simulink model "n98tot98reg60neu"  (R2023b)
settings: Solver=VariableStepAuto  StartTime=0.0  StopTime=10.0  RelTol=1e-3
libraries: neural x66
(part 2 of 3)

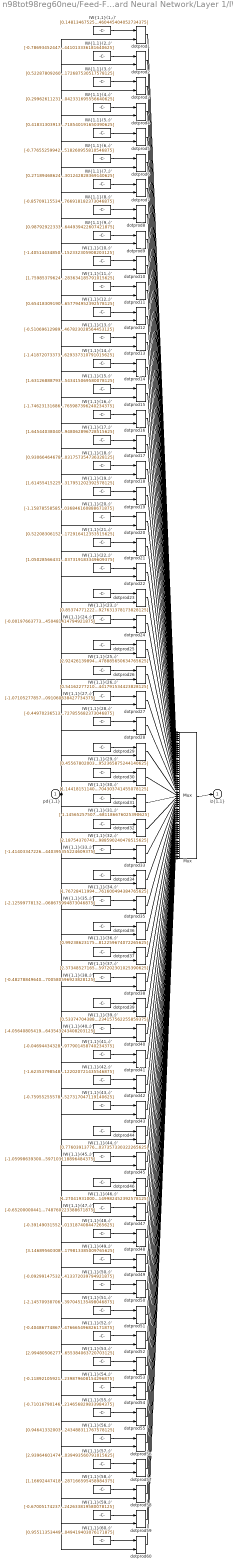
== system n98tot98reg60neu/Feed-Forward Neural Network/Layer 1/IW{1,1} ==
  "pd{1,1}" : Inport  PortDimensions=7
      mask Display: e = 0.06;c1 = [120 230 180]/255;c2 = ([120 230 180]+0)/(256+128);c3 = ([120 230 180]+128)/(256+128);patch([0 1 1 0],[0 0 1 1],c1);patch([0 1 1 1-e 1-e 0+e],[0 0 1 1-e 0+e 0+e],c2);patch([0 0 1 1-e 0+e 0+e],[0 1 1 1-e 1-e 0+e],c3);plot([0 1 1 0 0],[0 0 1 1 0]);
  "IW{1,1}(1,:)'" : Constant  Value=[0.1481346752533242161486981558482511900365352630615234375;0.98082353054952253756937352591194212436676025390625;-2.082918281795799853028938741772435605525970458984375;0.40694944026411672410858955117873847484588623046875;-1.0518399557692712509293642142438329756259918212890625;1.2557149846669120041298128853668458759784698486328125;-0.67808270069946752212075580246164463460445404052734375]
      mask Display: e = 0.06;c1 = [120 150 230]/255;c2 = ([120 150 230]+0)/383;c3 = ([120 150 230]+128)/383;patch([0 1 1 0],[0 0 1 1],c1);patch([0 1 1 1-e 1-e 0+e],[0 0 1 1-e 0+e 0+e],c2);patch([0 0 1 1-e 0+e 0+e],[0 1 1 1-e 1-e 0+e],c3);plot([0 1 1 0 0],[0 0 1 1 0]);disp('Weights');
  "IW{1,1}(10,:)'" : Constant  Value=[-1.4051443485085826079483695139060728251934051513671875;0.487311062264708161340109882075921632349491119384765625;-0.9939232561735884541320729113067500293254852294921875;0.69193945193100725443713372442289255559444427490234375;2.418400242942244648958194375154562294483184814453125;-3.03067098031489390308479414670728147029876708984375;-1.6729437161008047230126294380170293152332305908203125]
      mask Display: e = 0.06;c1 = [120 150 230]/255;c2 = ([120 150 230]+0)/383;c3 = ([120 150 230]+128)/383;patch([0 1 1 0],[0 0 1 1],c1);patch([0 1 1 1-e 1-e 0+e],[0 0 1 1-e 0+e 0+e],c2);patch([0 0 1 1-e 0+e 0+e],[0 1 1 1-e 1-e 0+e],c3);plot([0 1 1 0 0],[0 0 1 1 0]);disp('Weights');
  "IW{1,1}(11,:)'" : Constant  Value=[1.759853796240600676270560143166221678256988525390625;-0.55894441450671905613489798270165920257568359375;-1.4532069951682655695179846588871441781520843505859375;-1.18865973477518327428015254554338753223419189453125;0.89752928329863934653332080415566451847553253173828125;1.1526682692309073718917034057085402309894561767578125;-1.1487702266456720767706656260997988283634185791015625]
      mask Display: e = 0.06;c1 = [120 150 230]/255;c2 = ([120 150 230]+0)/383;c3 = ([120 150 230]+128)/383;patch([0 1 1 0],[0 0 1 1],c1);patch([0 1 1 1-e 1-e 0+e],[0 0 1 1-e 0+e 0+e],c2);patch([0 0 1 1-e 0+e 0+e],[0 1 1 1-e 1-e 0+e],c3);plot([0 1 1 0 0],[0 0 1 1 0]);disp('Weights');
  "IW{1,1}(12,:)'" : Constant  Value=[0.6541830919058633231344401792739517986774444580078125;-0.98785279841036466308423769078217446804046630859375;0.5520966690451316605248166524688713252544403076171875;-0.417983555830826636334762724800384603440761566162109375;-0.9204938395589810085084536694921553134918212890625;0.93854167778469499427984601425123400986194610595703125;-0.469771047647070283392878309314255602657794952392578125]
      mask Display: e = 0.06;c1 = [120 150 230]/255;c2 = ([120 150 230]+0)/383;c3 = ([120 150 230]+128)/383;patch([0 1 1 0],[0 0 1 1],c1);patch([0 1 1 1-e 1-e 0+e],[0 0 1 1-e 0+e 0+e],c2);patch([0 0 1 1-e 0+e 0+e],[0 1 1 1-e 1-e 0+e],c3);plot([0 1 1 0 0],[0 0 1 1 0]);disp('Weights');
  "IW{1,1}(13,:)'" : Constant  Value=[-0.51069612989874146879998306758352555334568023681640625;0.412856570783323884032967043822281993925571441650390625;0.397626390946691110617194908627425320446491241455078125;0.0344230577253679115301565616391599178314208984375;1.03739130513506427888614780385978519916534423828125;0.92439008882190598637151879302109591662883758544921875;0.03278356001701394906167053022727486677467823028564453125]
      mask Display: e = 0.06;c1 = [120 150 230]/255;c2 = ([120 150 230]+0)/383;c3 = ([120 150 230]+128)/383;patch([0 1 1 0],[0 0 1 1],c1);patch([0 1 1 1-e 1-e 0+e],[0 0 1 1-e 0+e 0+e],c2);patch([0 0 1 1-e 0+e 0+e],[0 1 1 1-e 1-e 0+e],c3);plot([0 1 1 0 0],[0 0 1 1 0]);disp('Weights');
  "IW{1,1}(14,:)'" : Constant  Value=[-1.4187207337306324550496583469794131815433502197265625;-0.431927417827714654752213618849054910242557525634765625;0.152434941407513291355968476636917330324649810791015625;-2.027428553931468702131724057835526764392852783203125;1.3251072881331922292957870013196952641010284423828125;0.6240741942748850856759190719458274543285369873046875;2.084603798637122196169002563692629337310791015625]
      mask Display: e = 0.06;c1 = [120 150 230]/255;c2 = ([120 150 230]+0)/383;c3 = ([120 150 230]+128)/383;patch([0 1 1 0],[0 0 1 1],c1);patch([0 1 1 1-e 1-e 0+e],[0 0 1 1-e 0+e 0+e],c2);patch([0 0 1 1-e 0+e 0+e],[0 1 1 1-e 1-e 0+e],c3);plot([0 1 1 0 0],[0 0 1 1 0]);disp('Weights');
  "IW{1,1}(15,:)'" : Constant  Value=[1.6312688879348937742719272137037478387355804443359375;-1.162534244233608848873018359881825745105743408203125;1.0284685549397938331139812362380325794219970703125;2.455316875408408261449721976532600820064544677734375;-2.869144685433620001191457049571909010410308837890625;1.3375400695654622307273484693723730742931365966796875;2.6889193919281684230782047961838543415069580078125]
      mask Display: e = 0.06;c1 = [120 150 230]/255;c2 = ([120 150 230]+0)/383;c3 = ([120 150 230]+128)/383;patch([0 1 1 0],[0 0 1 1],c1);patch([0 1 1 1-e 1-e 0+e],[0 0 1 1-e 0+e 0+e],c2);patch([0 0 1 1-e 0+e 0+e],[0 1 1 1-e 1-e 0+e],c3);plot([0 1 1 0 0],[0 0 1 1 0]);disp('Weights');
  "IW{1,1}(16,:)'" : Constant  Value=[-1.746231316863945171036220926907844841480255126953125;-1.15887605284371719704950010054744780063629150390625;0.50001076713111769489472635541460476815700531005859375;-2.84379068119553313209735279087908565998077392578125;0.129001045300250638536709857362438924610614776611328125;-1.0933162048887756778725588446832261979579925537109375;0.7263530548743071246775571125908754765987396240234375]
      mask Display: e = 0.06;c1 = [120 150 230]/255;c2 = ([120 150 230]+0)/383;c3 = ([120 150 230]+128)/383;patch([0 1 1 0],[0 0 1 1],c1);patch([0 1 1 1-e 1-e 0+e],[0 0 1 1-e 0+e 0+e],c2);patch([0 0 1 1-e 0+e 0+e],[0 1 1 1-e 1-e 0+e],c3);plot([0 1 1 0 0],[0 0 1 1 0]);disp('Weights');
  "IW{1,1}(17,:)'" : Constant  Value=[1.64544038040287698976271713036112487316131591796875;-3.633653677731499609393495120457373559474945068359375;-2.29787262698807293048730571172200143337249755859375;0.078067342091915847834826536200125701725482940673828125;-0.577295747878546539055832909070886671543121337890625;-1.619702917064653302503529630484990775585174560546875;1.7761068046404473452781758169294334948062896728515625]
      mask Display: e = 0.06;c1 = [120 150 230]/255;c2 = ([120 150 230]+0)/383;c3 = ([120 150 230]+128)/383;patch([0 1 1 0],[0 0 1 1],c1);patch([0 1 1 1-e 1-e 0+e],[0 0 1 1-e 0+e 0+e],c2);patch([0 0 1 1-e 0+e 0+e],[0 1 1 1-e 1-e 0+e],c3);plot([0 1 1 0 0],[0 0 1 1 0]);disp('Weights');
  "IW{1,1}(18,:)'" : Constant  Value=[0.93066464678121019193923757484299130737781524658203125;-1.9544287349273126164206360044772736728191375732421875;-1.023472620127600318795657585724256932735443115234375;0.98793022766258375977344030616222880780696868896484375;1.6281013571460698496906616128399036824703216552734375;-0.0185687723603052794174583794983846019022166728973388671875;-0.2930769639165078377374129559029825031757354736328125]
      mask Display: e = 0.06;c1 = [120 150 230]/255;c2 = ([120 150 230]+0)/383;c3 = ([120 150 230]+128)/383;patch([0 1 1 0],[0 0 1 1],c1);patch([0 1 1 1-e 1-e 0+e],[0 0 1 1-e 0+e 0+e],c2);patch([0 0 1 1-e 0+e 0+e],[0 1 1 1-e 1-e 0+e],c3);plot([0 1 1 0 0],[0 0 1 1 0]);disp('Weights');
  "IW{1,1}(19,:)'" : Constant  Value=[1.6145541522585509230935940649942494928836822509765625;0.91381367394026347117375053130672313272953033447265625;-0.371631548982591042307177531256456859409809112548828125;0.73502527154724550673137173362192697823047637939453125;1.5056615216127851031302498086006380617618560791015625;1.15739385289584983951272079139016568660736083984375;-1.45708523863142591636687939171679317951202392578125]
      mask Display: e = 0.06;c1 = [120 150 230]/255;c2 = ([120 150 230]+0)/383;c3 = ([120 150 230]+128)/383;patch([0 1 1 0],[0 0 1 1],c1);patch([0 1 1 1-e 1-e 0+e],[0 0 1 1-e 0+e 0+e],c2);patch([0 0 1 1-e 0+e 0+e],[0 1 1 1-e 1-e 0+e],c3);plot([0 1 1 0 0],[0 0 1 1 0]);disp('Weights');
  "IW{1,1}(2,:)'" : Constant  Value=[-0.7869345244760317381604863840038888156414031982421875;-0.346311954352809092672060842232895083725452423095703125;-1.556955762008559229769844023394398391246795654296875;-0.51529864332368091606184634656528942286968231201171875;0.868254630896831969266713713295757770538330078125;0.052275095673093983916768223707549623213708400726318359375;1.454283513794509818950473345466889441013336181640625]
      mask Display: e = 0.06;c1 = [120 150 230]/255;c2 = ([120 150 230]+0)/383;c3 = ([120 150 230]+128)/383;patch([0 1 1 0],[0 0 1 1],c1);patch([0 1 1 1-e 1-e 0+e],[0 0 1 1-e 0+e 0+e],c2);patch([0 0 1 1-e 0+e 0+e],[0 1 1 1-e 1-e 0+e],c3);plot([0 1 1 0 0],[0 0 1 1 0]);disp('Weights');
  "IW{1,1}(20,:)'" : Constant  Value=[-1.158785585859792188756500763702206313610076904296875;-0.9101893538308860609475914316135458648204803466796875;-0.2242153799095476240932356404300662688910961151123046875;4.6125770809612678391431472846306860446929931640625;-1.967721084439806755739255095249973237514495849609375;0.77232129956188710906417327350936830043792724609375;-0.07051684698582198762562001093101571314036846160888671875]
      mask Display: e = 0.06;c1 = [120 150 230]/255;c2 = ([120 150 230]+0)/383;c3 = ([120 150 230]+128)/383;patch([0 1 1 0],[0 0 1 1],c1);patch([0 1 1 1-e 1-e 0+e],[0 0 1 1-e 0+e 0+e],c2);patch([0 0 1 1-e 0+e 0+e],[0 1 1 1-e 1-e 0+e],c3);plot([0 1 1 0 0],[0 0 1 1 0]);disp('Weights');
  "IW{1,1}(21,:)'" : Constant  Value=[0.52208306152979744307884857335011474788188934326171875;-0.24553627119159637803846862880163826048374176025390625;0.74283311097407267453718304750509560108184814453125;-0.8132083009806365669902561421622522175312042236328125;-1.6353310904372870826506414232426322996616363525390625;0.804047841179728717264652004814706742763519287109375;0.30147537024770498792491935091675259172916412353515625]
      mask Display: e = 0.06;c1 = [120 150 230]/255;c2 = ([120 150 230]+0)/383;c3 = ([120 150 230]+128)/383;patch([0 1 1 0],[0 0 1 1],c1);patch([0 1 1 1-e 1-e 0+e],[0 0 1 1-e 0+e 0+e],c2);patch([0 0 1 1-e 0+e 0+e],[0 1 1 1-e 1-e 0+e],c3);plot([0 1 1 0 0],[0 0 1 1 0]);disp('Weights');
  "IW{1,1}(22,:)'" : Constant  Value=[1.050285664310628863660213028197176754474639892578125;-0.1436604121479605200573104184513795189559459686279296875;1.3658699547684276520698176682344637811183929443359375;-2.139623131427094815393274984671734273433685302734375;-0.476115789654785681594972857055836357176303863525390625;-2.445497663519104580842622453928925096988677978515625;-0.95852873762775236965438807601458393037319183349609375]
      mask Display: e = 0.06;c1 = [120 150 230]/255;c2 = ([120 150 230]+0)/383;c3 = ([120 150 230]+128)/383;patch([0 1 1 0],[0 0 1 1],c1);patch([0 1 1 1-e 1-e 0+e],[0 0 1 1-e 0+e 0+e],c2);patch([0 0 1 1-e 0+e 0+e],[0 1 1 1-e 1-e 0+e],c3);plot([0 1 1 0 0],[0 0 1 1 0]);disp('Weights');
  "IW{1,1}(23,:)'" : Constant  Value=[0.85374771222291812033944324866752140223979949951171875;1.4611201108056064423834641274879686534404754638671875;-0.71512999345489658420405021388432942330837249755859375;-1.5360765778745673060257104225456714630126953125;1.3057858257014036684751090433564968407154083251953125;-1.0436475254304660165161067197914235293865203857421875;1.2728096477339807535145155270583927631378173828125]
      mask Display: e = 0.06;c1 = [120 150 230]/255;c2 = ([120 150 230]+0)/383;c3 = ([120 150 230]+128)/383;patch([0 1 1 0],[0 0 1 1],c1);patch([0 1 1 1-e 1-e 0+e],[0 0 1 1-e 0+e 0+e],c2);patch([0 0 1 1-e 0+e 0+e],[0 1 1 1-e 1-e 0+e],c3);plot([0 1 1 0 0],[0 0 1 1 0]);disp('Weights');
  "IW{1,1}(24,:)'" : Constant  Value=[-0.0019766377326448647533396751896361820399761199951171875;-0.83118616146239043818155778353684581816196441650390625;0.373888659074529117187779547748505137860774993896484375;1.59975498434179375095709474408067762851715087890625;1.8936310356371277574538680710247717797756195068359375;-2.56484219821481662648920973879285156726837158203125;-0.73221593302772880473838768011773936450481414794921875]
      mask Display: e = 0.06;c1 = [120 150 230]/255;c2 = ([120 150 230]+0)/383;c3 = ([120 150 230]+128)/383;patch([0 1 1 0],[0 0 1 1],c1);patch([0 1 1 1-e 1-e 0+e],[0 0 1 1-e 0+e 0+e],c2);patch([0 0 1 1-e 0+e 0+e],[0 1 1 1-e 1-e 0+e],c3);plot([0 1 1 0 0],[0 0 1 1 0]);disp('Weights');
  "IW{1,1}(25,:)'" : Constant  Value=[2.924261398940739553609091672115027904510498046875;1.01135703353342254473545835935510694980621337890625;-0.40057513886989604134925002654199488461017608642578125;1.117845219342571194687252500443719327449798583984375;1.487336953128143068880717692081816494464874267578125;-0.3337818787676083420734585160971619188785552978515625;3.366286632630610231586842928663827478885650634765625]
      mask Display: e = 0.06;c1 = [120 150 230]/255;c2 = ([120 150 230]+0)/383;c3 = ([120 150 230]+128)/383;patch([0 1 1 0],[0 0 1 1],c1);patch([0 1 1 1-e 1-e 0+e],[0 0 1 1-e 0+e 0+e],c2);patch([0 0 1 1-e 0+e 0+e],[0 1 1 1-e 1-e 0+e],c3);plot([0 1 1 0 0],[0 0 1 1 0]);disp('Weights');
  "IW{1,1}(26,:)'" : Constant  Value=[0.54162277210162113050273546832613646984100341796875;0.456056013547237182326199445014935918152332305908203125;1.4394577727029942426639763652929104864597320556640625;0.58974019201134175727219144391710869967937469482421875;1.9862617127959680818349852415849454700946807861328125;0.291103928669838751819298749978770501911640167236328125;-2.381474711015628020760459548910148441791534423828125]
      mask Display: e = 0.06;c1 = [120 150 230]/255;c2 = ([120 150 230]+0)/383;c3 = ([120 150 230]+128)/383;patch([0 1 1 0],[0 0 1 1],c1);patch([0 1 1 1-e 1-e 0+e],[0 0 1 1-e 0+e 0+e],c2);patch([0 0 1 1-e 0+e 0+e],[0 1 1 1-e 1-e 0+e],c3);plot([0 1 1 0 0],[0 0 1 1 0]);disp('Weights');
  "IW{1,1}(27,:)'" : Constant  Value=[-1.071052778571999652967861038632690906524658203125;-2.02899035921602344245684435009025037288665771484375;-0.8560859121211625843983483719057403504848480224609375;0.59540640519818233133975127202575094997882843017578125;0.75214105415422505274136710795573890209197998046875;-0.43346848639706792027936899103224277496337890625;1.076762221099778482624742537154816091060638427734375]
      mask Display: e = 0.06;c1 = [120 150 230]/255;c2 = ([120 150 230]+0)/383;c3 = ([120 150 230]+128)/383;patch([0 1 1 0],[0 0 1 1],c1);patch([0 1 1 1-e 1-e 0+e],[0 0 1 1-e 0+e 0+e],c2);patch([0 0 1 1-e 0+e 0+e],[0 1 1 1-e 1-e 0+e],c3);plot([0 1 1 0 0],[0 0 1 1 0]);disp('Weights');
  "IW{1,1}(28,:)'" : Constant  Value=[-0.4497023651390212872769325258559547364711761474609375;-0.8805125386607233206603950748103670775890350341796875;-1.606489318533170784775165884639136493206024169921875;-1.447323751073491759910893961205147206783294677734375;1.3204566033571929484224938278202898800373077392578125;-0.1433022562635145880083342717625782825052738189697265625;-1.173633507304539858040470790001563727855682373046875]
      mask Display: e = 0.06;c1 = [120 150 230]/255;c2 = ([120 150 230]+0)/383;c3 = ([120 150 230]+128)/383;patch([0 1 1 0],[0 0 1 1],c1);patch([0 1 1 1-e 1-e 0+e],[0 0 1 1-e 0+e 0+e],c2);patch([0 0 1 1-e 0+e 0+e],[0 1 1 1-e 1-e 0+e],c3);plot([0 1 1 0 0],[0 0 1 1 0]);disp('Weights');
  "IW{1,1}(29,:)'" : Constant  Value=[0.455678020034327946330421355014550499618053436279296875;1.0449829035940758625855551144923083484172821044921875;-2.051400565385125940309762881952337920665740966796875;-2.269241494744366871572083255159668624401092529296875;4.0322839793207787550954890321008861064910888671875;0.80328637261176349948499364472809247672557830810546875;4.19454985578971051296548466780222952365875244140625]
      mask Display: e = 0.06;c1 = [120 150 230]/255;c2 = ([120 150 230]+0)/383;c3 = ([120 150 230]+128)/383;patch([0 1 1 0],[0 0 1 1],c1);patch([0 1 1 1-e 1-e 0+e],[0 0 1 1-e 0+e 0+e],c2);patch([0 0 1 1-e 0+e 0+e],[0 1 1 1-e 1-e 0+e],c3);plot([0 1 1 0 0],[0 0 1 1 0]);disp('Weights');
  "IW{1,1}(3,:)'" : Constant  Value=[0.52287809260233941710538374536554329097270965576171875;0.355086158017595965308288441519835032522678375244140625;0.3211806987072407526540018807281740009784698486328125;-0.172433039949836774962221852547372691333293914794921875;-0.02907109420287723455800232841284014284610748291015625;-0.936005019789345027447780012153089046478271484375;1.1683911275902467696852227163617499172687530517578125]
      mask Display: e = 0.06;c1 = [120 150 230]/255;c2 = ([120 150 230]+0)/383;c3 = ([120 150 230]+128)/383;patch([0 1 1 0],[0 0 1 1],c1);patch([0 1 1 1-e 1-e 0+e],[0 0 1 1-e 0+e 0+e],c2);patch([0 0 1 1-e 0+e 0+e],[0 1 1 1-e 1-e 0+e],c3);plot([0 1 1 0 0],[0 0 1 1 0]);disp('Weights');
  "IW{1,1}(30,:)'" : Constant  Value=[1.1441815114008682119361992590711452066898345947265625;0.02635002074122540227651967370547936297953128814697265625;1.1697060189576917732523497761576436460018157958984375;-2.07603958112650044398606041795574128627777099609375;-1.523338123097244700687724616727791726589202880859375;1.2813465289053180828915401434642262756824493408203125;-0.301678114240235828447111998684704303741455078125]
      mask Display: e = 0.06;c1 = [120 150 230]/255;c2 = ([120 150 230]+0)/383;c3 = ([120 150 230]+128)/383;patch([0 1 1 0],[0 0 1 1],c1);patch([0 1 1 1-e 1-e 0+e],[0 0 1 1-e 0+e 0+e],c2);patch([0 0 1 1-e 0+e 0+e],[0 1 1 1-e 1-e 0+e],c3);plot([0 1 1 0 0],[0 0 1 1 0]);disp('Weights');
  "IW{1,1}(31,:)'" : Constant  Value=[-1.1456525750787356354720714080031029880046844482421875;-0.301316378862511335956497759980265982449054718017578125;-0.6999713143398993420163378686993382871150970458984375;-1.888670407036998621919110519229434430599212646484375;-0.51493465015129358253176405924023129045963287353515625;1.09374415185767315250586761976592242717742919921875;-1.172688349926057416183766690664924681186676025390625]
      mask Display: e = 0.06;c1 = [120 150 230]/255;c2 = ([120 150 230]+0)/383;c3 = ([120 150 230]+128)/383;patch([0 1 1 0],[0 0 1 1],c1);patch([0 1 1 1-e 1-e 0+e],[0 0 1 1-e 0+e 0+e],c2);patch([0 0 1 1-e 0+e 0+e],[0 1 1 1-e 1-e 0+e],c3);plot([0 1 1 0 0],[0 0 1 1 0]);disp('Weights');
  "IW{1,1}(32,:)'" : Constant  Value=[2.187543707432160200454518417245708405971527099609375;0.7832629532967370078466728955390863120555877685546875;0.97277406417956502338029167731292545795440673828125;0.169364411870373654522836659452877938747406005859375;-0.1872178173399863532200271265537594445049762725830078125;-1.635072077562477854684175326838158071041107177734375;0.0374795167828784470120950800264836288988590240478515625]
      mask Display: e = 0.06;c1 = [120 150 230]/255;c2 = ([120 150 230]+0)/383;c3 = ([120 150 230]+128)/383;patch([0 1 1 0],[0 0 1 1],c1);patch([0 1 1 1-e 1-e 0+e],[0 0 1 1-e 0+e 0+e],c2);patch([0 0 1 1-e 0+e 0+e],[0 1 1 1-e 1-e 0+e],c3);plot([0 1 1 0 0],[0 0 1 1 0]);disp('Weights');
  "IW{1,1}(33,:)'" : Constant  Value=[-1.4140334722618492779844245887943543493747711181640625;-1.066226188394075347076750404085032641887664794921875;-0.74303173177076786704020605611731298267841339111328125;0.59865982615122026455622972207493148744106292724609375;-0.46737583966662021861537823497201316058635711669921875;-0.145915447642352480439598139128065668046474456787109375;0.6450607346262733354791407691664062440395355224609375]
      mask Display: e = 0.06;c1 = [120 150 230]/255;c2 = ([120 150 230]+0)/383;c3 = ([120 150 230]+128)/383;patch([0 1 1 0],[0 0 1 1],c1);patch([0 1 1 1-e 1-e 0+e],[0 0 1 1-e 0+e 0+e],c2);patch([0 0 1 1-e 0+e 0+e],[0 1 1 1-e 1-e 0+e],c3);plot([0 1 1 0 0],[0 0 1 1 0]);disp('Weights');
  "IW{1,1}(34,:)'" : Constant  Value=[1.767284119945664588868794453446753323078155517578125;-0.6493741207138825632938505805213935673236846923828125;-0.255236564518358355346805410590604878962039947509765625;-2.13669533467837791107513112365268170833587646484375;0.80266841289320833841003377528977580368518829345703125;0.61122329910277761744197277948842383921146392822265625;-0.5399939366629686876564164776937104761600494384765625]
      mask Display: e = 0.06;c1 = [120 150 230]/255;c2 = ([120 150 230]+0)/383;c3 = ([120 150 230]+128)/383;patch([0 1 1 0],[0 0 1 1],c1);patch([0 1 1 1-e 1-e 0+e],[0 0 1 1-e 0+e 0+e],c2);patch([0 0 1 1-e 0+e 0+e],[0 1 1 1-e 1-e 0+e],c3);plot([0 1 1 0 0],[0 0 1 1 0]);disp('Weights');
  "IW{1,1}(35,:)'" : Constant  Value=[-2.12599778132206562730743826250545680522918701171875;1.3608125008815721290744704674580134451389312744140625;-0.7325358825414862717906316902372054755687713623046875;0.240060365986900781098967172511038370430469512939453125;0.18982699817795001262510368178482167422771453857421875;-1.0066882538136978642029362163157202303409576416015625;0.667860286161154004247464399668388068675994873046875]
      mask Display: e = 0.06;c1 = [120 150 230]/255;c2 = ([120 150 230]+0)/383;c3 = ([120 150 230]+128)/383;patch([0 1 1 0],[0 0 1 1],c1);patch([0 1 1 1-e 1-e 0+e],[0 0 1 1-e 0+e 0+e],c2);patch([0 0 1 1-e 0+e 0+e],[0 1 1 1-e 1-e 0+e],c3);plot([0 1 1 0 0],[0 0 1 1 0]);disp('Weights');
  "IW{1,1}(36,:)'" : Constant  Value=[0.992386231759784909201016489532776176929473876953125;-0.10079863677393478826882500243300455622375011444091796875;-0.89913155892687812720254214582382701337337493896484375;-1.153666025787317916950769358663819730281829833984375;0.186564489102124586583641985271242447197437286376953125;2.13673253963647180597718033823184669017791748046875;2.591152548548058209831879139528609812259674072265625]
      mask Display: e = 0.06;c1 = [120 150 230]/255;c2 = ([120 150 230]+0)/383;c3 = ([120 150 230]+128)/383;patch([0 1 1 0],[0 0 1 1],c1);patch([0 1 1 1-e 1-e 0+e],[0 0 1 1-e 0+e 0+e],c2);patch([0 0 1 1-e 0+e 0+e],[0 1 1 1-e 1-e 0+e],c3);plot([0 1 1 0 0],[0 0 1 1 0]);disp('Weights');
  "IW{1,1}(37,:)'" : Constant  Value=[2.373485271659477202632615444599650800228118896484375;-2.83140944472043454283038954599760472774505615234375;-0.2381591970668265056954027159008546732366085052490234375;1.6073649182960274561793312386726029217243194580078125;0.1270632058802902975003235042095184326171875;-0.290937777914213047125713273999281227588653564453125;2.903333553776429543091808227472938597202301025390625]
      mask Display: e = 0.06;c1 = [120 150 230]/255;c2 = ([120 150 230]+0)/383;c3 = ([120 150 230]+128)/383;patch([0 1 1 0],[0 0 1 1],c1);patch([0 1 1 1-e 1-e 0+e],[0 0 1 1-e 0+e 0+e],c2);patch([0 0 1 1-e 0+e 0+e],[0 1 1 1-e 1-e 0+e],c3);plot([0 1 1 0 0],[0 0 1 1 0]);disp('Weights');
  "IW{1,1}(38,:)'" : Constant  Value=[-0.482788496408222689293410212485468946397304534912109375;1.6104028950399194020093318613362498581409454345703125;-1.865988325170027994914789815084077417850494384765625;0.75686623013146536731454716573352925479412078857421875;0.803638662707797823969713135738857090473175048828125;-0.624867558425080016348829303751699626445770263671875;0.73596606492041971581130610502441413700580596923828125]
      mask Display: e = 0.06;c1 = [120 150 230]/255;c2 = ([120 150 230]+0)/383;c3 = ([120 150 230]+128)/383;patch([0 1 1 0],[0 0 1 1],c1);patch([0 1 1 1-e 1-e 0+e],[0 0 1 1-e 0+e 0+e],c2);patch([0 0 1 1-e 0+e 0+e],[0 1 1 1-e 1-e 0+e],c3);plot([0 1 1 0 0],[0 0 1 1 0]);disp('Weights');
  "IW{1,1}(39,:)'" : Constant  Value=[0.5337470438813813888856429912266321480274200439453125;0.84274856967459876866399781647487543523311614990234375;-1.95409080267971635436197175295092165470123291015625;0.42544403042022604921612582984380424022674560546875;0.9690675152028200844966931981616653501987457275390625;0.0163222485195519372014327785791465430520474910736083984375;-0.491484984158165827405895242918631993234157562255859375]
      mask Display: e = 0.06;c1 = [120 150 230]/255;c2 = ([120 150 230]+0)/383;c3 = ([120 150 230]+128)/383;patch([0 1 1 0],[0 0 1 1],c1);patch([0 1 1 1-e 1-e 0+e],[0 0 1 1-e 0+e 0+e],c2);patch([0 0 1 1-e 0+e 0+e],[0 1 1 1-e 1-e 0+e],c3);plot([0 1 1 0 0],[0 0 1 1 0]);disp('Weights');
  "IW{1,1}(4,:)'" : Constant  Value=[0.299626112316270176716415107875945977866649627685546875;-0.044314293017502691396369840504121384583413600921630859375;-0.8841463713183135286755032211658544838428497314453125;0.7744232725463380262453938485123217105865478515625;1.8909629644727130592940511633059941232204437255859375;0.062323560497111706035777700662947609089314937591552734375;-0.11719207511177499869692297806977876462042331695556640625]
      mask Display: e = 0.06;c1 = [120 150 230]/255;c2 = ([120 150 230]+0)/383;c3 = ([120 150 230]+128)/383;patch([0 1 1 0],[0 0 1 1],c1);patch([0 1 1 1-e 1-e 0+e],[0 0 1 1-e 0+e 0+e],c2);patch([0 0 1 1-e 0+e 0+e],[0 1 1 1-e 1-e 0+e],c3);plot([0 1 1 0 0],[0 0 1 1 0]);disp('Weights');
  "IW{1,1}(40,:)'" : Constant  Value=[-4.05640805419469785420005791820585727691650390625;0.0873765616747470830194544078040053136646747589111328125;0.54901834404562188662879407274886034429073333740234375;0.89968084756964561421455073286779224872589111328125;1.7184637967256561896789435195387341082096099853515625;-1.3935197143518334161882421540212817490100860595703125;-2.623692509614226953118532037478871643543243408203125]
      mask Display: e = 0.06;c1 = [120 150 230]/255;c2 = ([120 150 230]+0)/383;c3 = ([120 150 230]+128)/383;patch([0 1 1 0],[0 0 1 1],c1);patch([0 1 1 1-e 1-e 0+e],[0 0 1 1-e 0+e 0+e],c2);patch([0 0 1 1-e 0+e 0+e],[0 1 1 1-e 1-e 0+e],c3);plot([0 1 1 0 0],[0 0 1 1 0]);disp('Weights');
  "IW{1,1}(41,:)'" : Constant  Value=[-0.046944343288031924188441479373068432323634624481201171875;-2.21537331420981953300497480086050927639007568359375;-1.2718477750401888659581572937895543873310089111328125;0.2532434280552477989800763680250383913516998291015625;-0.38837008773848669118677889855462126433849334716796875;1.0430562979632067577284715298446826636791229248046875;-0.92779194210217408311791587038896977901458740234375]
      mask Display: e = 0.06;c1 = [120 150 230]/255;c2 = ([120 150 230]+0)/383;c3 = ([120 150 230]+128)/383;patch([0 1 1 0],[0 0 1 1],c1);patch([0 1 1 1-e 1-e 0+e],[0 0 1 1-e 0+e 0+e],c2);patch([0 0 1 1-e 0+e 0+e],[0 1 1 1-e 1-e 0+e],c3);plot([0 1 1 0 0],[0 0 1 1 0]);disp('Weights');
  "IW{1,1}(42,:)'" : Constant  Value=[-1.6235379854818445810593630085350014269351959228515625;0.98250437107865373764781224963371641933917999267578125;1.90239772700385589843108391505666077136993408203125;0.3618940465058153588273626155569218099117279052734375;0.311560429313485542923700677420129068195819854736328125;2.113010718428258716272694073268212378025054931640625;-0.08559181635963357404062179512038710527122020721435546875]
      mask Display: e = 0.06;c1 = [120 150 230]/255;c2 = ([120 150 230]+0)/383;c3 = ([120 150 230]+128)/383;patch([0 1 1 0],[0 0 1 1],c1);patch([0 1 1 1-e 1-e 0+e],[0 0 1 1-e 0+e 0+e],c2);patch([0 0 1 1-e 0+e 0+e],[0 1 1 1-e 1-e 0+e],c3);plot([0 1 1 0 0],[0 0 1 1 0]);disp('Weights');
  "IW{1,1}(43,:)'" : Constant  Value=[-0.75955255578861358145559279364533722400665283203125;1.3921115451136893970129904118948616087436676025390625;0.438296223731076184382260407801368273794651031494140625;-0.78872599627513484410457067497191019356250762939453125;-1.7965397122145831954043160294531844556331634521484375;0.41442701575381268863651484934962354600429534912109375;-0.7917432291391934828794774148263968527317047119140625]
      mask Display: e = 0.06;c1 = [120 150 230]/255;c2 = ([120 150 230]+0)/383;c3 = ([120 150 230]+128)/383;patch([0 1 1 0],[0 0 1 1],c1);patch([0 1 1 1-e 1-e 0+e],[0 0 1 1-e 0+e 0+e],c2);patch([0 0 1 1-e 0+e 0+e],[0 1 1 1-e 1-e 0+e],c3);plot([0 1 1 0 0],[0 0 1 1 0]);disp('Weights');
  "IW{1,1}(44,:)'" : Constant  Value=[0.77603913776969035698272136869491077959537506103515625;1.68618633989586275134797688224352896213531494140625;-0.0668610125904696150911377117154188454151153564453125;-0.54391986928281832458509370553656481206417083740234375;-1.628652778124873190535026878933422267436981201171875;1.319361974881373189560918035567738115787506103515625;-1.025986300680023166620458141551353037357330322265625]
      mask Display: e = 0.06;c1 = [120 150 230]/255;c2 = ([120 150 230]+0)/383;c3 = ([120 150 230]+128)/383;patch([0 1 1 0],[0 0 1 1],c1);patch([0 1 1 1-e 1-e 0+e],[0 0 1 1-e 0+e 0+e],c2);patch([0 0 1 1-e 0+e 0+e],[0 1 1 1-e 1-e 0+e],c3);plot([0 1 1 0 0],[0 0 1 1 0]);disp('Weights');
  "IW{1,1}(45,:)'" : Constant  Value=[-1.059986393001422388948640218586660921573638916015625;-0.173101130652922263752913067946792580187320709228515625;0.5844790773023811336628341450705192983150482177734375;-1.4850851960119795247550200656405650079250335693359375;-2.491597453765368896938525722362101078033447265625;-0.69934109868302651857874252527835778892040252685546875;-0.9044014878802657531053910133778117597103118896484375]
      mask Display: e = 0.06;c1 = [120 150 230]/255;c2 = ([120 150 230]+0)/383;c3 = ([120 150 230]+128)/383;patch([0 1 1 0],[0 0 1 1],c1);patch([0 1 1 1-e 1-e 0+e],[0 0 1 1-e 0+e 0+e],c2);patch([0 0 1 1-e 0+e 0+e],[0 1 1 1-e 1-e 0+e],c3);plot([0 1 1 0 0],[0 0 1 1 0]);disp('Weights');
  "IW{1,1}(46,:)'" : Constant  Value=[1.2704193100027347806957322973175905644893646240234375;0.36762899058214071335015660224598832428455352783203125;1.2338475706229130590685372226289473474025726318359375;1.61977613534372721915133297443389892578125;1.4297303052058583094918731148936785757541656494140625;1.009376369554987551424574121483601629734039306640625;-1.5254997695976364457948193376068957149982452392578125]
      mask Display: e = 0.06;c1 = [120 150 230]/255;c2 = ([120 150 230]+0)/383;c3 = ([120 150 230]+128)/383;patch([0 1 1 0],[0 0 1 1],c1);patch([0 1 1 1-e 1-e 0+e],[0 0 1 1-e 0+e 0+e],c2);patch([0 0 1 1-e 0+e 0+e],[0 1 1 1-e 1-e 0+e],c3);plot([0 1 1 0 0],[0 0 1 1 0]);disp('Weights');
  "IW{1,1}(47,:)'" : Constant  Value=[-0.6520000044181470943982503740699030458927154541015625;-2.14807689392080902734960545785725116729736328125;0.30508269178191227410934516228735446929931640625;1.4101409733411525149193721517804078757762908935546875;0.86058815026270452097634233723510988056659698486328125;0.56656820153376930004895939418929629027843475341796875;0.503688223996419548456060510943643748760223388671875]
      mask Display: e = 0.06;c1 = [120 150 230]/255;c2 = ([120 150 230]+0)/383;c3 = ([120 150 230]+128)/383;patch([0 1 1 0],[0 0 1 1],c1);patch([0 1 1 1-e 1-e 0+e],[0 0 1 1-e 0+e 0+e],c2);patch([0 0 1 1-e 0+e 0+e],[0 1 1 1-e 1-e 0+e],c3);plot([0 1 1 0 0],[0 0 1 1 0]);disp('Weights');
  "IW{1,1}(48,:)'" : Constant  Value=[-0.391490315520112763802984545691288076341152191162109375;-0.1411084660676686919345002024783752858638763427734375;1.215498247946994236912132691941224038600921630859375;-0.01961802326384708139439538854276179336011409759521484375;3.85616003720454525449667926295660436153411865234375;0.52960589523922207977335574469179846346378326416015625;-0.977924126398966198081552647636272013187408447265625]
      mask Display: e = 0.06;c1 = [120 150 230]/255;c2 = ([120 150 230]+0)/383;c3 = ([120 150 230]+128)/383;patch([0 1 1 0],[0 0 1 1],c1);patch([0 1 1 1-e 1-e 0+e],[0 0 1 1-e 0+e 0+e],c2);patch([0 0 1 1-e 0+e 0+e],[0 1 1 1-e 1-e 0+e],c3);plot([0 1 1 0 0],[0 0 1 1 0]);disp('Weights');
  "IW{1,1}(49,:)'" : Constant  Value=[3.146895603083233794450279674492776393890380859375;1.7472349608462358627747335049207322299480438232421875;0.7900047284623408216930329217575490474700927734375;-0.4267675030149826742587038097553886473178863525390625;-1.165080190804833382145488940295763313770294189453125;0.71233753204131355918349299827241338789463043212890625;-1.6692508500826639394887251910404302179813385009765625]
      mask Display: e = 0.06;c1 = [120 150 230]/255;c2 = ([120 150 230]+0)/383;c3 = ([120 150 230]+128)/383;patch([0 1 1 0],[0 0 1 1],c1);patch([0 1 1 1-e 1-e 0+e],[0 0 1 1-e 0+e 0+e],c2);patch([0 0 1 1-e 0+e 0+e],[0 1 1 1-e 1-e 0+e],c3);plot([0 1 1 0 0],[0 0 1 1 0]);disp('Weights');
  "IW{1,1}(5,:)'" : Constant  Value=[0.418313039130509434215809960733167827129364013671875;0.59154140343533090362626580827054567635059356689453125;1.52828163417684503855298316921107470989227294921875;-1.3352094420734068602740762798930518329143524169921875;-0.1773906306009228883713291224921704269945621490478515625;-0.9304403197455177743080412255949340760707855224609375;-0.521077102426085847497461145394481718540191650390625]
      mask Display: e = 0.06;c1 = [120 150 230]/255;c2 = ([120 150 230]+0)/383;c3 = ([120 150 230]+128)/383;patch([0 1 1 0],[0 0 1 1],c1);patch([0 1 1 1-e 1-e 0+e],[0 0 1 1-e 0+e 0+e],c2);patch([0 0 1 1-e 0+e 0+e],[0 1 1 1-e 1-e 0+e],c3);plot([0 1 1 0 0],[0 0 1 1 0]);disp('Weights');
  "IW{1,1}(50,:)'" : Constant  Value=[-0.09299147532523883985522417106039938516914844512939453125;0.2212028814998839021388477021901053376495838165283203125;-1.367502038876399428346530839917249977588653564453125;0.149462870458643148907640352263115346431732177734375;1.43803812210721648767730584950186312198638916015625;-0.56873955080151816776634632333298213779926300048828125;-0.418886678529261480274925588673795573413372039794921875]
      mask Display: e = 0.06;c1 = [120 150 230]/255;c2 = ([120 150 230]+0)/383;c3 = ([120 150 230]+128)/383;patch([0 1 1 0],[0 0 1 1],c1);patch([0 1 1 1-e 1-e 0+e],[0 0 1 1-e 0+e 0+e],c2);patch([0 0 1 1-e 0+e 0+e],[0 1 1 1-e 1-e 0+e],c3);plot([0 1 1 0 0],[0 0 1 1 0]);disp('Weights');
  "IW{1,1}(51,:)'" : Constant  Value=[-2.14570938706170455390065399114973843097686767578125;-0.91149469900424351376244658240466378629207611083984375;0.8098365880171394248776550739421509206295013427734375;1.512309897695889748803210750338621437549591064453125;-0.2119992648588315820035177239333279430866241455078125;-1.0326483768972087862181297168717719614505767822265625;-0.85290627225207937822659687299164943397045135498046875]
      mask Display: e = 0.06;c1 = [120 150 230]/255;c2 = ([120 150 230]+0)/383;c3 = ([120 150 230]+128)/383;patch([0 1 1 0],[0 0 1 1],c1);patch([0 1 1 1-e 1-e 0+e],[0 0 1 1-e 0+e 0+e],c2);patch([0 0 1 1-e 0+e 0+e],[0 1 1 1-e 1-e 0+e],c3);plot([0 1 1 0 0],[0 0 1 1 0]);disp('Weights');
  "IW{1,1}(52,:)'" : Constant  Value=[-0.404867748676235150728786038598627783358097076416015625;-0.42029731151777582898176888193120248615741729736328125;1.299408072829371096901240889565087854862213134765625;1.2308012084313804113122614580788649618625640869140625;0.80657817399877862474255607594386674463748931884765625;-0.4344717411564300579840391947072930634021759033203125;-0.55894690716519235262893516846816055476665496826171875]
      mask Display: e = 0.06;c1 = [120 150 230]/255;c2 = ([120 150 230]+0)/383;c3 = ([120 150 230]+128)/383;patch([0 1 1 0],[0 0 1 1],c1);patch([0 1 1 1-e 1-e 0+e],[0 0 1 1-e 0+e 0+e],c2);patch([0 0 1 1-e 0+e 0+e],[0 1 1 1-e 1-e 0+e],c3);plot([0 1 1 0 0],[0 0 1 1 0]);disp('Weights');
  "IW{1,1}(53,:)'" : Constant  Value=[2.994805062774202664144240770838223397731781005859375;0.00956422219174242298211918722472546505741775035858154296875;-1.8875362364771504086746745088021270930767059326171875;1.17653478225301366677513215108774602413177490234375;-2.8280186048595368220048840157687664031982421875;-0.9560636326461084966155112851993180811405181884765625;1.286147465360354846808377260458655655384063720703125]
      mask Display: e = 0.06;c1 = [120 150 230]/255;c2 = ([120 150 230]+0)/383;c3 = ([120 150 230]+128)/383;patch([0 1 1 0],[0 0 1 1],c1);patch([0 1 1 1-e 1-e 0+e],[0 0 1 1-e 0+e 0+e],c2);patch([0 0 1 1-e 0+e 0+e],[0 1 1 1-e 1-e 0+e],c3);plot([0 1 1 0 0],[0 0 1 1 0]);disp('Weights');
  "IW{1,1}(54,:)'" : Constant  Value=[-0.11892105921896745091004277128376998007297515869140625;-0.03155636073634802973852941931909299455583095550537109375;0.56303231191200120431261666453792713582515716552734375;-3.230346520504300489307070165523327887058258056640625;-0.13754832481948586764275432869908399879932403564453125;0.393691138460503908813592488513677380979061126708984375;0.33788978981991402150697467732243239879608154296875]
      mask Display: e = 0.06;c1 = [120 150 230]/255;c2 = ([120 150 230]+0)/383;c3 = ([120 150 230]+128)/383;patch([0 1 1 0],[0 0 1 1],c1);patch([0 1 1 1-e 1-e 0+e],[0 0 1 1-e 0+e 0+e],c2);patch([0 0 1 1-e 0+e 0+e],[0 1 1 1-e 1-e 0+e],c3);plot([0 1 1 0 0],[0 0 1 1 0]);disp('Weights');
  "IW{1,1}(55,:)'" : Constant  Value=[-0.71016790146078145884445120827876962721347808837890625;1.0935467362190263163057579731685109436511993408203125;1.272018505730863058289514810894615948200225830078125;-1.0273503440232898409334438838413916528224945068359375;-0.7905594533536899337633485629339702427387237548828125;0.04351703972455667202012818961520679295063018798828125;1.0257073066875166400535590582876466214656829833984375]
      mask Display: e = 0.06;c1 = [120 150 230]/255;c2 = ([120 150 230]+0)/383;c3 = ([120 150 230]+128)/383;patch([0 1 1 0],[0 0 1 1],c1);patch([0 1 1 1-e 1-e 0+e],[0 0 1 1-e 0+e 0+e],c2);patch([0 0 1 1-e 0+e 0+e],[0 1 1 1-e 1-e 0+e],c3);plot([0 1 1 0 0],[0 0 1 1 0]);disp('Weights');
  "IW{1,1}(56,:)'" : Constant  Value=[0.946413320038624217289680018438957631587982177734375;1.249286020237861283277425172855146229267120361328125;0.851543212870219168308949519996531307697296142578125;-0.58110211253185595214887371184886433184146881103515625;-0.057464275041770963847742592633949243463575839996337890625;-1.5361770938010093079384432712686248123645782470703125;0.70097584625887698894786126402323134243488311767578125]
      mask Display: e = 0.06;c1 = [120 150 230]/255;c2 = ([120 150 230]+0)/383;c3 = ([120 150 230]+128)/383;patch([0 1 1 0],[0 0 1 1],c1);patch([0 1 1 1-e 1-e 0+e],[0 0 1 1-e 0+e 0+e],c2);patch([0 0 1 1-e 0+e 0+e],[0 1 1 1-e 1-e 0+e],c3);plot([0 1 1 0 0],[0 0 1 1 0]);disp('Weights');
  "IW{1,1}(57,:)'" : Constant  Value=[2.939646014749645264174660042044706642627716064453125;1.1119041572133898654328731936402618885040283203125;0.1584816358570919903048235255482723005115985870361328125;0.58868485646394319577012765876133926212787628173828125;0.9076904121541866654609975739731453359127044677734375;0.02702888780874730667580507770253461785614490509033203125;-0.5897681905720251194225056678988039493560791015625]
      mask Display: e = 0.06;c1 = [120 150 230]/255;c2 = ([120 150 230]+0)/383;c3 = ([120 150 230]+128)/383;patch([0 1 1 0],[0 0 1 1],c1);patch([0 1 1 1-e 1-e 0+e],[0 0 1 1-e 0+e 0+e],c2);patch([0 0 1 1-e 0+e 0+e],[0 1 1 1-e 1-e 0+e],c3);plot([0 1 1 0 0],[0 0 1 1 0]);disp('Weights');
  "IW{1,1}(58,:)'" : Constant  Value=[1.1669244741818076693817829436738975346088409423828125;0.46734753031421438773662657695240341126918792724609375;-0.2521107756519402887107617061701603233814239501953125;1.1788154623263127351862067371257580816745758056640625;1.4261259702778972258130352201987989246845245361328125;1.01116418999620094609781517647206783294677734375;-0.482824972350044789859424554379074834287166595458984375]
      mask Display: e = 0.06;c1 = [120 150 230]/255;c2 = ([120 150 230]+0)/383;c3 = ([120 150 230]+128)/383;patch([0 1 1 0],[0 0 1 1],c1);patch([0 1 1 1-e 1-e 0+e],[0 0 1 1-e 0+e 0+e],c2);patch([0 0 1 1-e 0+e 0+e],[0 1 1 1-e 1-e 0+e],c3);plot([0 1 1 0 0],[0 0 1 1 0]);disp('Weights');
  "IW{1,1}(59,:)'" : Constant  Value=[-0.67005174237528486447246223178808577358722686767578125;-1.3332691048322085070054754396551288664340972900390625;-0.08006667081900807614314174998071393929421901702880859375;-0.65479307717354096052275735928560607135295867919921875;-2.304252998455214918038791438448242843151092529296875;-0.08909511595894002711215620138318627141416072845458984375;-0.62333896748935579967820785896037705242633819580078125]
      mask Display: e = 0.06;c1 = [120 150 230]/255;c2 = ([120 150 230]+0)/383;c3 = ([120 150 230]+128)/383;patch([0 1 1 0],[0 0 1 1],c1);patch([0 1 1 1-e 1-e 0+e],[0 0 1 1-e 0+e 0+e],c2);patch([0 0 1 1-e 0+e 0+e],[0 1 1 1-e 1-e 0+e],c3);plot([0 1 1 0 0],[0 0 1 1 0]);disp('Weights');
  "IW{1,1}(6,:)'" : Constant  Value=[-0.77655259942523435778838347687269560992717742919921875;-1.9785985975969950789732365592499263584613800048828125;1.51717872626245497968966446933336555957794189453125;-0.84923223416891546744267316171317361295223236083984375;-1.9660353975579358820624520376441068947315216064453125;2.908312985613832779563381336629390716552734375;-0.7290988528125221801445832170429639518260955810546875]
      mask Display: e = 0.06;c1 = [120 150 230]/255;c2 = ([120 150 230]+0)/383;c3 = ([120 150 230]+128)/383;patch([0 1 1 0],[0 0 1 1],c1);patch([0 1 1 1-e 1-e 0+e],[0 0 1 1-e 0+e 0+e],c2);patch([0 0 1 1-e 0+e 0+e],[0 1 1 1-e 1-e 0+e],c3);plot([0 1 1 0 0],[0 0 1 1 0]);disp('Weights');
  "IW{1,1}(60,:)'" : Constant  Value=[0.9551135344970955731724870929610915482044219970703125;1.29909791522576245625941737671382725238800048828125;0.57115029795468996720586574156186543405055999755859375;-1.9264376234658886488659845781512558460235595703125;1.204663511903115047374512869282625615596771240234375;-0.83513430005156708002544974078773520886898040771484375;1.12902403733098832816494905273430049419403076171875]
      mask Display: e = 0.06;c1 = [120 150 230]/255;c2 = ([120 150 230]+0)/383;c3 = ([120 150 230]+128)/383;patch([0 1 1 0],[0 0 1 1],c1);patch([0 1 1 1-e 1-e 0+e],[0 0 1 1-e 0+e 0+e],c2);patch([0 0 1 1-e 0+e 0+e],[0 1 1 1-e 1-e 0+e],c3);plot([0 1 1 0 0],[0 0 1 1 0]);disp('Weights');
  "IW{1,1}(7,:)'" : Constant  Value=[0.27189468624378287930909436909132637083530426025390625;3.629852733769265427099526277743279933929443359375;0.70251120641849695847014345417846925556659698486328125;0.60038807473390576330274370775441639125347137451171875;-0.134506423642610395408070189660065807402133941650390625;-0.52709940237550634289931394960149191319942474365234375;-2.641200353812040990675313878455199301242828369140625]
      mask Display: e = 0.06;c1 = [120 150 230]/255;c2 = ([120 150 230]+0)/383;c3 = ([120 150 230]+128)/383;patch([0 1 1 0],[0 0 1 1],c1);patch([0 1 1 1-e 1-e 0+e],[0 0 1 1-e 0+e 0+e],c2);patch([0 0 1 1-e 0+e 0+e],[0 1 1 1-e 1-e 0+e],c3);plot([0 1 1 0 0],[0 0 1 1 0]);disp('Weights');
  "IW{1,1}(8,:)'" : Constant  Value=[-0.85709115534920365941928821484907530248165130615234375;1.9584471118207125162058446221635676920413970947265625;-1.5397194471680075711361723733716644346714019775390625;-0.53003260320531409011124424068839289247989654541015625;-0.420637138818104217019566704038879834115505218505859375;0.1706433782406077404036892630756483413279056549072265625;-1.44030447599171207428980778786353766918182373046875]
      mask Display: e = 0.06;c1 = [120 150 230]/255;c2 = ([120 150 230]+0)/383;c3 = ([120 150 230]+128)/383;patch([0 1 1 0],[0 0 1 1],c1);patch([0 1 1 1-e 1-e 0+e],[0 0 1 1-e 0+e 0+e],c2);patch([0 0 1 1-e 0+e 0+e],[0 1 1 1-e 1-e 0+e],c3);plot([0 1 1 0 0],[0 0 1 1 0]);disp('Weights');
  "IW{1,1}(9,:)'" : Constant  Value=[0.98792922333648203192524306359700858592987060546875;-1.8924015713870694366249836093629710376262664794921875;0.331150537867130390079495327881886623799800872802734375;-0.027921316171867237299064612443544319830834865570068359375;0.349316352390757145496280600127647630870342254638671875;0.70591388934536947186160205092164687812328338623046875;-0.51969307978539880377155668611521832644939422607421875]
      mask Display: e = 0.06;c1 = [120 150 230]/255;c2 = ([120 150 230]+0)/383;c3 = ([120 150 230]+128)/383;patch([0 1 1 0],[0 0 1 1],c1);patch([0 1 1 1-e 1-e 0+e],[0 0 1 1-e 0+e 0+e],c2);patch([0 0 1 1-e 0+e 0+e],[0 1 1 1-e 1-e 0+e],c3);plot([0 1 1 0 0],[0 0 1 1 0]);disp('Weights');
  Mux : Mux  Inputs=60
      mask Display: e = 0.06;c1 = [120 150 230]/255;c2 = ([120 150 230]+0)/383;c3 = ([120 150 230]+128)/383;patch([0 1 1 0],[0 0 1 1],c1);patch([0 1 1 1-e 1-e 0+e],[0 0 1 1-e 0+e 0+e],c2);patch([0 0 1 1-e 0+e 0+e],[0 1 1 1-e 1-e 0+e],c3);plot([0 1 1 0 0],[0 0 1 1 0]);disp('Mux');
  dotprod{1..60} (60 alike) : neural/Weight Functions/dotprod
  "iz{1,1}" : Outport
      mask Display: e = 0.06;c1 = [120 230 180]/255;c2 = ([120 230 180]+0)/(256+128);c3 = ([120 230 180]+128)/(256+128);patch([0 1 1 0],[0 0 1 1],c1);patch([0 1 1 1-e 1-e 0+e],[0 0 1 1-e 0+e 0+e],c2);patch([0 0 1 1-e 0+e 0+e],[0 1 1 1-e 1-e 0+e],c3);plot([0 1 1 0 0],[0 0 1 1 0]);
  wires:
  "IW{1,1}(1,:)'"/1 -> dotprod1/1
  "pd{1,1}"/1 -> dotprod1/2, dotprod2/2, dotprod3/2, dotprod4/2, dotprod5/2, dotprod6/2, dotprod7/2, dotprod8/2, dotprod9/2, dotprod10/2, dotprod11/2, dotprod12/2, dotprod13/2, dotprod14/2, dotprod15/2, dotprod16/2, dotprod17/2, dotprod18/2, dotprod19/2, dotprod20/2, dotprod21/2, dotprod22/2, dotprod23/2, dotprod24/2, dotprod25/2, dotprod26/2, dotprod27/2, dotprod28/2, dotprod29/2, dotprod30/2, dotprod31/2, dotprod32/2, dotprod33/2, dotprod34/2, dotprod35/2, dotprod36/2, dotprod37/2, dotprod38/2, dotprod39/2, dotprod40/2, dotprod41/2, dotprod42/2, dotprod43/2, dotprod44/2, dotprod45/2, dotprod46/2, dotprod47/2, dotprod48/2, dotprod49/2, dotprod50/2, dotprod51/2, dotprod52/2, dotprod53/2, dotprod54/2, dotprod55/2, dotprod56/2, dotprod57/2, dotprod58/2, dotprod59/2, dotprod60/2
  dotprod1/1 -> Mux/1
  "IW{1,1}(2,:)'"/1 -> dotprod2/1
  dotprod2/1 -> Mux/2
  "IW{1,1}(3,:)'"/1 -> dotprod3/1
  dotprod3/1 -> Mux/3
  "IW{1,1}(4,:)'"/1 -> dotprod4/1
  dotprod4/1 -> Mux/4
  "IW{1,1}(5,:)'"/1 -> dotprod5/1
  dotprod5/1 -> Mux/5
  "IW{1,1}(6,:)'"/1 -> dotprod6/1
  dotprod6/1 -> Mux/6
  "IW{1,1}(7,:)'"/1 -> dotprod7/1
  dotprod7/1 -> Mux/7
  "IW{1,1}(8,:)'"/1 -> dotprod8/1
  dotprod8/1 -> Mux/8
  "IW{1,1}(9,:)'"/1 -> dotprod9/1
  dotprod9/1 -> Mux/9
  "IW{1,1}(10,:)'"/1 -> dotprod10/1
  dotprod10/1 -> Mux/10
  "IW{1,1}(11,:)'"/1 -> dotprod11/1
  dotprod11/1 -> Mux/11
  "IW{1,1}(12,:)'"/1 -> dotprod12/1
  dotprod12/1 -> Mux/12
  "IW{1,1}(13,:)'"/1 -> dotprod13/1
  dotprod13/1 -> Mux/13
  "IW{1,1}(14,:)'"/1 -> dotprod14/1
  dotprod14/1 -> Mux/14
  "IW{1,1}(15,:)'"/1 -> dotprod15/1
  dotprod15/1 -> Mux/15
  "IW{1,1}(16,:)'"/1 -> dotprod16/1
  dotprod16/1 -> Mux/16
  "IW{1,1}(17,:)'"/1 -> dotprod17/1
  dotprod17/1 -> Mux/17
  "IW{1,1}(18,:)'"/1 -> dotprod18/1
  dotprod18/1 -> Mux/18
  "IW{1,1}(19,:)'"/1 -> dotprod19/1
  dotprod19/1 -> Mux/19
  "IW{1,1}(20,:)'"/1 -> dotprod20/1
  dotprod20/1 -> Mux/20
  "IW{1,1}(21,:)'"/1 -> dotprod21/1
  dotprod21/1 -> Mux/21
  "IW{1,1}(22,:)'"/1 -> dotprod22/1
  dotprod22/1 -> Mux/22
  "IW{1,1}(23,:)'"/1 -> dotprod23/1
  dotprod23/1 -> Mux/23
  "IW{1,1}(24,:)'"/1 -> dotprod24/1
  dotprod24/1 -> Mux/24
  "IW{1,1}(25,:)'"/1 -> dotprod25/1
  dotprod25/1 -> Mux/25
  "IW{1,1}(26,:)'"/1 -> dotprod26/1
  dotprod26/1 -> Mux/26
  "IW{1,1}(27,:)'"/1 -> dotprod27/1
  dotprod27/1 -> Mux/27
  "IW{1,1}(28,:)'"/1 -> dotprod28/1
  dotprod28/1 -> Mux/28
  "IW{1,1}(29,:)'"/1 -> dotprod29/1
  dotprod29/1 -> Mux/29
  "IW{1,1}(30,:)'"/1 -> dotprod30/1
  dotprod30/1 -> Mux/30
  "IW{1,1}(31,:)'"/1 -> dotprod31/1
  dotprod31/1 -> Mux/31
  "IW{1,1}(32,:)'"/1 -> dotprod32/1
  dotprod32/1 -> Mux/32
  "IW{1,1}(33,:)'"/1 -> dotprod33/1
  dotprod33/1 -> Mux/33
  "IW{1,1}(34,:)'"/1 -> dotprod34/1
  dotprod34/1 -> Mux/34
  "IW{1,1}(35,:)'"/1 -> dotprod35/1
  dotprod35/1 -> Mux/35
  "IW{1,1}(36,:)'"/1 -> dotprod36/1
  dotprod36/1 -> Mux/36
  "IW{1,1}(37,:)'"/1 -> dotprod37/1
  dotprod37/1 -> Mux/37
  "IW{1,1}(38,:)'"/1 -> dotprod38/1
  dotprod38/1 -> Mux/38
  "IW{1,1}(39,:)'"/1 -> dotprod39/1
  dotprod39/1 -> Mux/39
  "IW{1,1}(40,:)'"/1 -> dotprod40/1
  dotprod40/1 -> Mux/40
  "IW{1,1}(41,:)'"/1 -> dotprod41/1
  dotprod41/1 -> Mux/41
  "IW{1,1}(42,:)'"/1 -> dotprod42/1
  dotprod42/1 -> Mux/42
  "IW{1,1}(43,:)'"/1 -> dotprod43/1
  dotprod43/1 -> Mux/43
  "IW{1,1}(44,:)'"/1 -> dotprod44/1
  dotprod44/1 -> Mux/44
  "IW{1,1}(45,:)'"/1 -> dotprod45/1
  dotprod45/1 -> Mux/45
  "IW{1,1}(46,:)'"/1 -> dotprod46/1
  dotprod46/1 -> Mux/46
  "IW{1,1}(47,:)'"/1 -> dotprod47/1
  dotprod47/1 -> Mux/47
  "IW{1,1}(48,:)'"/1 -> dotprod48/1
  dotprod48/1 -> Mux/48
  "IW{1,1}(49,:)'"/1 -> dotprod49/1
  dotprod49/1 -> Mux/49
  "IW{1,1}(50,:)'"/1 -> dotprod50/1
  dotprod50/1 -> Mux/50
  "IW{1,1}(51,:)'"/1 -> dotprod51/1
  dotprod51/1 -> Mux/51
  "IW{1,1}(52,:)'"/1 -> dotprod52/1
  dotprod52/1 -> Mux/52
  "IW{1,1}(53,:)'"/1 -> dotprod53/1
  dotprod53/1 -> Mux/53
  "IW{1,1}(54,:)'"/1 -> dotprod54/1
  dotprod54/1 -> Mux/54
  "IW{1,1}(55,:)'"/1 -> dotprod55/1
  dotprod55/1 -> Mux/55
  "IW{1,1}(56,:)'"/1 -> dotprod56/1
  dotprod56/1 -> Mux/56
  "IW{1,1}(57,:)'"/1 -> dotprod57/1
  dotprod57/1 -> Mux/57
  "IW{1,1}(58,:)'"/1 -> dotprod58/1
  dotprod58/1 -> Mux/58
  "IW{1,1}(59,:)'"/1 -> dotprod59/1
  dotprod59/1 -> Mux/59
  "IW{1,1}(60,:)'"/1 -> dotprod60/1
  dotprod60/1 -> Mux/60
  Mux/1 -> "iz{1,1}"/1

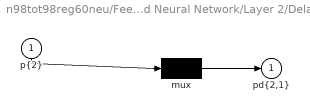
== system n98tot98reg60neu/Feed-Forward Neural Network/Layer 2/Delays 1 ==
  "p{2}" : Inport  PortDimensions=60
      mask Display: e = 0.06;c1 = [120 230 180]/255;c2 = ([120 230 180]+0)/(256+128);c3 = ([120 230 180]+128)/(256+128);patch([0 1 1 0],[0 0 1 1],c1);patch([0 1 1 1-e 1-e 0+e],[0 0 1 1-e 0+e 0+e],c2);patch([0 0 1 1-e 0+e 0+e],[0 1 1 1-e 1-e 0+e],c3);plot([0 1 1 0 0],[0 0 1 1 0]);
  mux : Mux  Inputs=1
      mask Display: e = 0.06;c1 = [120 150 230]/255;c2 = ([120 150 230]+0)/383;c3 = ([120 150 230]+128)/383;patch([0 1 1 0],[0 0 1 1],c1);patch([0 1 1 1-e 1-e 0+e],[0 0 1 1-e 0+e 0+e],c2);patch([0 0 1 1-e 0+e 0+e],[0 1 1 1-e 1-e 0+e],c3);plot([0 1 1 0 0],[0 0 1 1 0]);disp('Mux')
  "pd{2,1}" : Outport
      mask Display: e = 0.06;c1 = [120 230 180]/255;c2 = ([120 230 180]+0)/(256+128);c3 = ([120 230 180]+128)/(256+128);patch([0 1 1 0],[0 0 1 1],c1);patch([0 1 1 1-e 1-e 0+e],[0 0 1 1-e 0+e 0+e],c2);patch([0 0 1 1-e 0+e 0+e],[0 1 1 1-e 1-e 0+e],c3);plot([0 1 1 0 0],[0 0 1 1 0]);
  wires:
  "p{2}"/1 -> mux/1
  mux/1 -> "pd{2,1}"/1
